simulink subsystem "controllerSSNominalReducedOrderObserver"  (R2024b)
settings: Solver=VariableStepAuto  StartTime=0.0  StopTime=10.0  RelTol=1e-3
values from neighbouring files (symbols this model uses):
  K_stateFB = place(sigmaD.A, sigmaD.B, [discrete_lambda1,discrete_lambda2])    [Controller_SS_direct_design_control_vars.m]
  Nu = solution(3,:)    [Controller_SS_direct_design_control_vars.m]
  Nx = solution(1:2,:)    [Controller_SS_direct_design_control_vars.m]
settings Model: Creator=Utente  LastModifiedBy=Buton

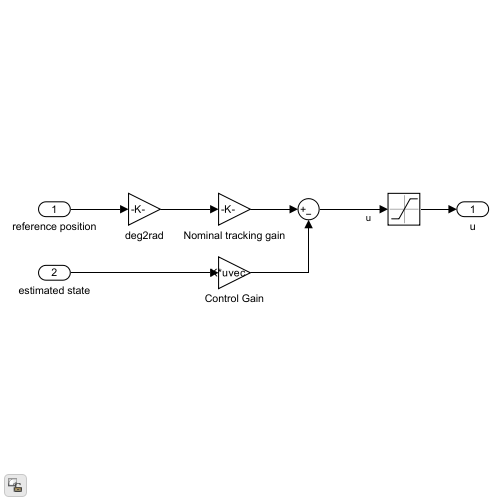
[thumbnail: Simulink's stored preview of the top-level diagram]
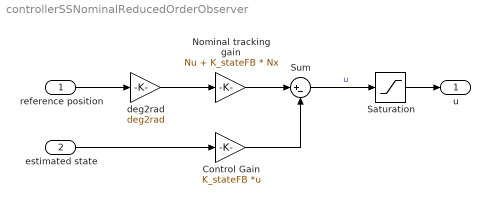
== system controllerSSNominalReducedOrderObserver ==
  reference position : Inport
  estimated state : Inport  Port=2
  Control Gain : Gain  Gain=K_stateFB  Multiplication=Matrix(K*u) (u vector)
  Nominal tracking gain : Gain  Gain=Nu + K_stateFB * Nx
  Saturation : Saturate  UpperLimit=12  LowerLimit=-12
  Sum : Sum  Inputs=|+-
  deg2rad : Gain  Gain=deg2rad
  u : Outport
  wires:
  estimated state/1 -> Control Gain/1
  reference position/1 -> deg2rad/1
  Nominal tracking gain/1 -> Sum/1
  Control Gain/1 -> Sum/2
  Sum/1 -> Saturation/1  "u"
  deg2rad/1 -> Nominal tracking gain/1
  Saturation/1 -> u/1
